simulink model "sync_boost"  (R2023b)
settings: Solver=VariableStepAuto  StartTime=0.0  StopTime=1  RelTol=1e-3
libraries: spsCurrentMeasurementLib x4, spsSeriesRLCBranchLib x4, spsVoltageMeasurementLib x4, spsMosfetLib x2, spsDCVoltageSourceLib x1, sps_lib x1
settings Model: Creator=23227  LastModifiedBy=23227

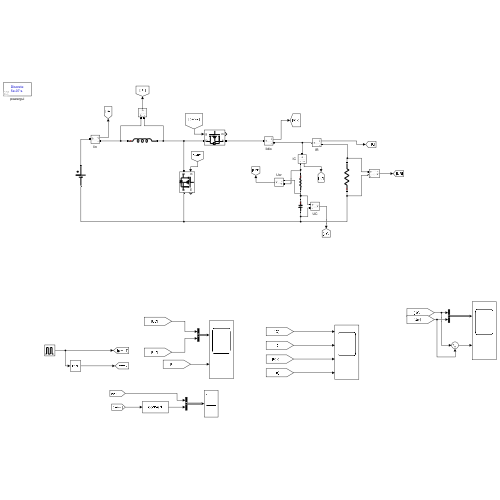
[thumbnail: Simulink's stored preview of the top-level diagram]
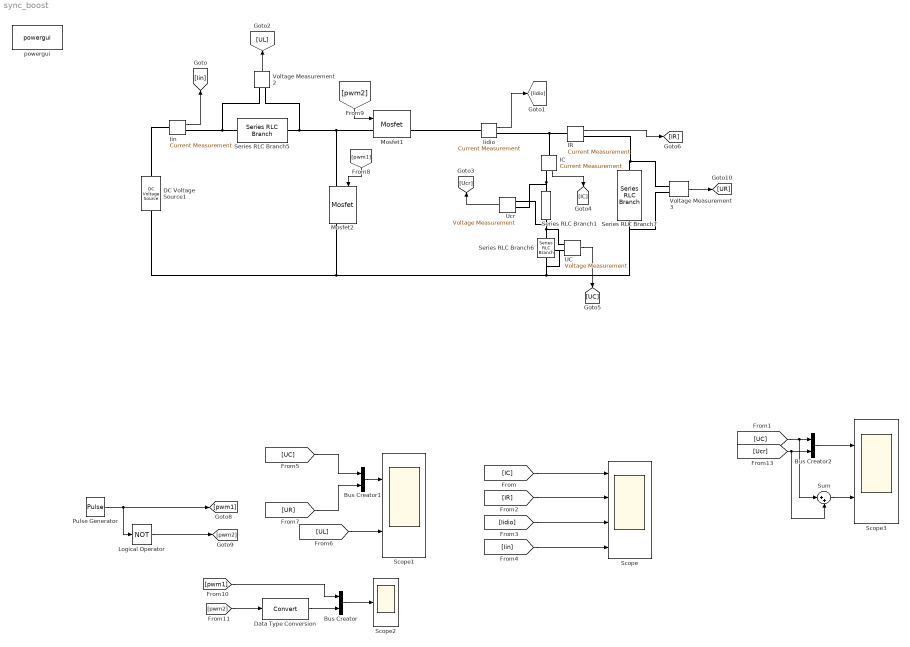
== system sync_boost ==
  Bus Creator : BusCreator  Inputs=2
  Bus Creator1 : BusCreator  Inputs=2
  Bus Creator2 : BusCreator  Inputs=2
  DC Voltage Source1 : spsDCVoltageSourceLib/DC Voltage Source  Amplitude=48  Measurements=None
  Data Type Conversion : DataTypeConversion  SaturateOnIntegerOverflow=off  RndMeth=Floor
  IC : spsCurrentMeasurementLib/Current Measurement  PhasorSimulation=off  OutputType=Complex  PSBequivalent=0
  IR : spsCurrentMeasurementLib/Current Measurement  PhasorSimulation=off  OutputType=Complex  PSBequivalent=0
  Iidio : spsCurrentMeasurementLib/Current Measurement  PhasorSimulation=off  OutputType=Complex  PSBequivalent=0
  Iin : spsCurrentMeasurementLib/Current Measurement  PhasorSimulation=off  OutputType=Complex  PSBequivalent=0
  Logical Operator : Logic  Operator=NOT  AllPortsSameDT=off  OutDataTypeStr=boolean
  Mosfet1 : spsMosfetLib/Mosfet  Ron=0.1  Lon=0  Rd=0.00001  Vfd=0  IC=0  Rs=1e5  Cs=inf  Measurements=on
  Mosfet2 : spsMosfetLib/Mosfet  Ron=0.1  Lon=0  Rd=0.00001  Vfd=0  IC=0  Rs=1e5  Cs=inf  Measurements=on
  Pulse Generator : DiscretePulseGenerator  PulseType=Time based  Period=1/20e3  PulseWidth=50
  Scope : Scope  NumInputPorts=4
  Scope1 : Scope  NumInputPorts=2
  Scope2 : Scope
  Scope3 : Scope  NumInputPorts=2
  Series RLC Branch1 : spsSeriesRLCBranchLib/Series RLC Branch  LConnTagsString=__new0  RConnTagsString=__new0  BranchType=R  Resistance=8.696e-3  Inductance=1e-3  SetiL0=off  InitialCurrent=0  Capacitance=4.5e-4  Setx0=off  InitialVoltage=0  Measurements=None
  Series RLC Branch5 : spsSeriesRLCBranchLib/Series RLC Branch  LConnTagsString=__new0  RConnTagsString=__new0  BranchType=L  Resistance=1  Inductance=2.2e-3  SetiL0=off  InitialCurrent=0  Capacitance=1e-6  Setx0=off  InitialVoltage=0  Measurements=None
  Series RLC Branch6 : spsSeriesRLCBranchLib/Series RLC Branch  LConnTagsString=__new0  RConnTagsString=__new0  BranchType=C  Resistance=1  Inductance=1e-3  SetiL0=off  InitialCurrent=0  Capacitance=1.725e-3  Setx0=off  InitialVoltage=0  Measurements=None
  Series RLC Branch7 : spsSeriesRLCBranchLib/Series RLC Branch  LConnTagsString=__new0  RConnTagsString=__new0  BranchType=R  Resistance=2.4  Inductance=1e-3  SetiL0=off  InitialCurrent=0  Capacitance=1e-6  Setx0=off  InitialVoltage=0  Measurements=None
  Sum : Sum  Inputs=|++
  UC : spsVoltageMeasurementLib/Voltage Measurement  PhasorSimulation=off  OutputType=Complex  PSBequivalent=0
  Ucr : spsVoltageMeasurementLib/Voltage Measurement  PhasorSimulation=off  OutputType=Complex  PSBequivalent=0
  Voltage Measurement2 : spsVoltageMeasurementLib/Voltage Measurement  PhasorSimulation=off  OutputType=Complex  PSBequivalent=0
  Voltage Measurement3 : spsVoltageMeasurementLib/Voltage Measurement  PhasorSimulation=off  OutputType=Complex  PSBequivalent=0
  powergui : sps_lib/powergui  Priority=1  SimulationMode=Discrete  SampleTime=1/20e3/100  frequency=60  Iterations=50  frequencyindice=0  Pbase=100e6  ErrMax=1e-4  UnitsV=kV  UnitsW=MW  buscounter=0  FunctionMessages=off  echomessages=off  EnableUseOfTLC=off  CurrentSourceSwitches=off  DisableSnubberDevices=off  DisableRonSwitches=off  DisableVfSwitches=off  DisplayEquations=off  AutomaticDiscreteSolvers=off  SolverType=Tustin/Backward Euler (TBE)  Interpol=off  ExternalGateDelay=off  methode=off  Ts=100  x0status=blocks  SPID=on  SwTol=0  HookPort=off  NonlinearTolerance=1e-4  nMaxIteration=100  ContinueOnMaxIteration=off  RestoreLinks=warning  ResistiveCurrentMeasurement=off  Frange=[0:2:500]  Ylog=off  Xlog=on  ShowGrid=off  save=off  variable=ZData  structure=0  ZoomFFT=off  StartTime=0.0  cycles=1  DisplayStyle=1  fundamental=60  FreqAxis=off  MaxFrequency=1000  frequencyindicesteady=1  RmsSteady=1  display=off
  wires:
  [pwm1] -> Bus Creator/1
  Data Type Conversion/1 -> Bus Creator/2
  [UC] -> Bus Creator1/1
  IR/1 -> [IR]
  [UL] -> Scope1/2
  [UR] -> Bus Creator1/2
  Pulse Generator/1 -> Logical Operator/1, [pwm1]
  [Iidio] -> Scope/3
  [IC] -> Scope/1
  IC/1 -> [IC]
  Voltage Measurement2/1 -> [UL]
  Logical Operator/1 -> [pwm2]
  Iidio/1 -> [Iidio]
  Iin/1 -> [Iin]
  [Iin] -> Scope/4
  [pwm2] -> Data Type Conversion/1
  Bus Creator/1 -> Scope2/1
  UC/1 -> [UC]
  [IR] -> Scope/2
  [pwm1] -> Mosfet2/1
  Voltage Measurement3/1 -> [UR]
  [pwm2] -> Mosfet1/1
  Bus Creator1/1 -> Scope1/1
  Ucr/1 -> [Ucr]
  Bus Creator2/1 -> Scope3/1
  [Ucr] -> Sum/2, Bus Creator2/2
  [UC] -> Sum/1, Bus Creator2/1
  Sum/1 -> Scope3/2
  connections:
  Series RLC Branch5/LConn1 -- Iin/RConn1 -- Voltage Measurement2/LConn1
  Mosfet2/LConn1 -- Mosfet1/LConn1 -- Voltage Measurement2/LConn2 -- Series RLC Branch5/RConn1
  DC Voltage Source1/LConn1 -- Voltage Measurement3/LConn2 -- Series RLC Branch7/LConn1 -- UC/LConn2 -- Series RLC Branch6/RConn1 -- Mosfet2/RConn1
  Series RLC Branch6/LConn1 -- Ucr/LConn2 -- Series RLC Branch1/RConn1 -- UC/LConn1
  DC Voltage Source1/RConn1 -- Iin/LConn1
  Mosfet1/RConn1 -- Iidio/LConn1
  IC/LConn1 -- IR/LConn1 -- Iidio/RConn1
  Voltage Measurement3/LConn1 -- IR/RConn1 -- Series RLC Branch7/RConn1
  IC/RConn1 -- Ucr/LConn1 -- Series RLC Branch1/LConn1
